simulink model "TubeMPC"  (Simulink 9.1)
settings: Solver=VariableStepAuto  StartTime=0.0  StopTime=40  FixedStep=0.1  RelTol=1e-3
undefined symbols (not defined in the file): ck_all, cx_all, cy_all, cyaw_all
libraries: Solver_SF x1, simulink x1
settings Model: Creator=MaoWenJie  LastModifiedBy=MaoWenJie
settings DataIOCC: SaveFormat=Dataset
settings OptimizationCC: LifeSpan=auto
settings DebuggingCC: UnderspecifiedInitializationDetection=Simplified  MergeDetectMultiDrivingBlocksExec=error  SFUnexpectedBacktrackingDiag=error  SFNoUnconditionalDefaultTransitionDiag=error  SFExecutionAtInitializationDiag=warning
settings HardwareCC: ProdBitPerPointer=64  ProdBitPerSizeT=64  ProdBitPerPtrDiffT=64  ProdLargestAtomicFloat=Float  ProdIntDivRoundTo=Zero  ProdEndianess=LittleEndian  ProdWordSize=64  ProdHWDeviceType=Intel->x86-64 (Windows64)
settings ModelReferenceCC: PropagateSignalLabelsOutOfModel=on
settings CodeAppCC: StateflowObjectComments=off
settings GRTTargetCC: TargetLangStandard=C99 (ISO)  CombineOutputUpdateFcns=on  GRTInterface=off
settings ConfigComp: CovMetricSettings=dwe  CovHtmlReporting=off  CovSaveCumulativeToWorkspaceVar=off  CovSaveSingleToWorkspaceVar=off  CovExternalEMLEnable=on

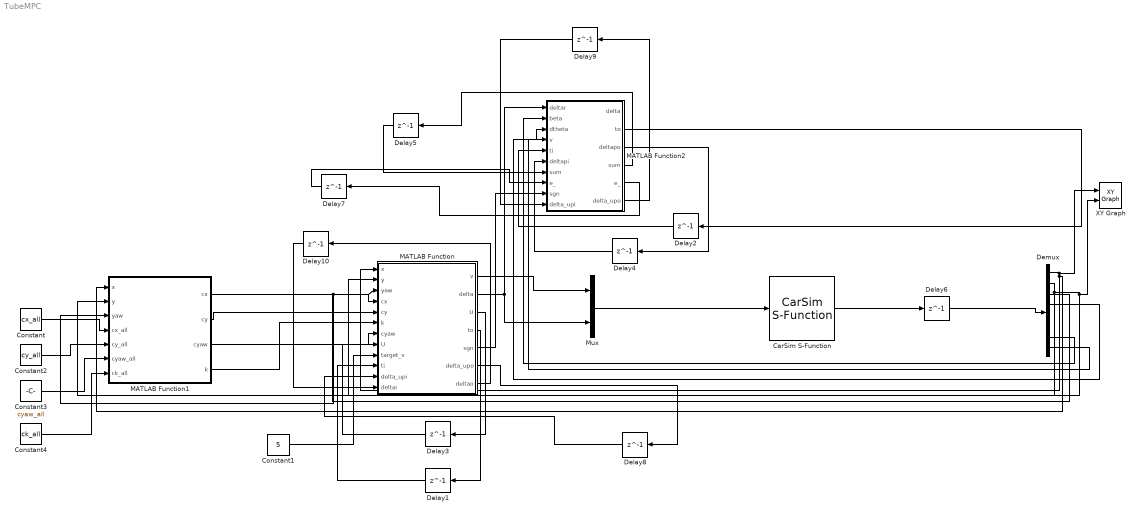
== system TubeMPC ==
  CarSim S-Function : Solver_SF/CarSim S-Function  Priority=3  SIMFILE=simfile.sim
  Constant : Constant  Value=cx_all
  Constant1 : Constant  Value=5
  Constant2 : Constant  Value=cy_all
  Constant3 : Constant  Value=cyaw_all
  Constant4 : Constant  Value=ck_all
  Delay{1..10} (10 alike) : Delay  DelayLength=1  InitialCondition=0
  Demux : Demux  Outputs=8
  MATLAB Function : MATLAB Function  Priority=2  InitFcn=|  TreatAsAtomicUnit=on
      | x = 0.1; y = -0.1; yaw = 0.1; 
      | U = [0.01;0.01];cx = 0.1;cy = -0.1;k = 1;cyaw = 1;ti = 0;
      | t = 0;
  MATLAB Function1 : MATLAB Function  Priority=1  TreatAsAtomicUnit=on
  MATLAB Function2 : MATLAB Function  InitFcn=ti = 0;deltapi = 0  TreatAsAtomicUnit=on
  Mux : Mux  Inputs=2
  XY Graph : simulink/Sinks/XY Graph  xmin=-1  xmax=200  ymin=-4  ymax=5  st=-1
  wires:
  Constant4/1 -> MATLAB Function1/7(ck_all)
  Constant3/1 -> MATLAB Function1/6(cyaw_all)
  Delay3/1 -> MATLAB Function/8("U ")
  Constant2/1 -> MATLAB Function1/5(cy_all)
  MATLAB Function1/1(cx) -> MATLAB Function/4(cx)
  MATLAB Function1/3(cyaw) -> MATLAB Function/7(cyaw)
  MATLAB Function/3(U) -> Delay3/1
  Constant/1 -> MATLAB Function1/4(cx_all)
  MATLAB Function1/4(k) -> MATLAB Function/6(k)
  Constant1/1 -> MATLAB Function/9(target_v)
  MATLAB Function1/2(cy) -> MATLAB Function/5(cy)
  CarSim S-Function/1 -> Delay6/1
  Delay6/1 -> Demux/1
  Demux/1 -> XY Graph/1, MATLAB Function1/1(x), MATLAB Function/1(x)
  Demux/2 -> XY Graph/2, MATLAB Function1/2(y), MATLAB Function/2(y)
  Demux/3 -> MATLAB Function1/3(yaw), MATLAB Function/3(yaw)
  MATLAB Function/1(v) -> Mux/1
  Mux/1 -> CarSim S-Function/1
  MATLAB Function/4(to) -> Delay1/1
  Delay1/1 -> MATLAB Function/10(ti)
  MATLAB Function/2(delta) -> Mux/2, MATLAB Function2/1(deltar)
  Demux/7 -> MATLAB Function2/2(beta)
  Demux/8 -> MATLAB Function2/3(dtheta)
  Demux/4 -> MATLAB Function2/4(v)
  MATLAB Function2/2(to) -> Delay2/1
  Delay2/1 -> MATLAB Function2/5(ti)
  MATLAB Function2/3(deltapo) -> Delay4/1
  Delay4/1 -> MATLAB Function2/6(deltapi)
  MATLAB Function2/4(sum) -> Delay5/1
  Delay5/1 -> MATLAB Function2/7("sum ")
  MATLAB Function2/5(e_) -> Delay7/1
  Delay7/1 -> MATLAB Function2/8("e_ ")
  MATLAB Function/5(sgn) -> MATLAB Function2/9(sgn)
  MATLAB Function/6(delta_upo) -> Delay8/1
  Delay8/1 -> MATLAB Function/11(delta_upi)
  MATLAB Function2/6(delta_upo) -> Delay9/1
  Delay9/1 -> MATLAB Function2/10(delta_upi)
  MATLAB Function/7(deltao) -> Delay10/1
  Delay10/1 -> MATLAB Function/12(deltai)

== matlab function MATLAB Function ==
  data: v output double; x input double; delta output double; y input double; yaw input double; cx input double; cy input double; k input double; cyaw input double; U input double size=2; target_v input double; U output double; ti input double; to output double; sgn output double; delta_upi input double; delta_upo output double; deltai input double; deltao output double
function    [v,delta,U,to,sgn,delta_upo,deltao] = ...
    tubeMpc_control(x,y,yaw,cx,cy,k,cyaw,U,target_v,ti,delta_upi,deltai) 
coder.extrinsic('dlqr');
coder.extrinsic('optimoptions');
coder.extrinsic('quadprog');
Length = 2.6;
yaw = yaw*pi/180;
u = [x,y,yaw];
vd1=target_v ;
vd2=atan(Length * k);
dt = 0.4;



if ti == 0
r = [cx, cy, cyaw];
    Nx=3;%状态量的个数
    Nu =2;%控制量的个数
    Np =60;%预测步长
    Nc=30;%控制步长
    Row=10;%松弛因子
    Q=100*eye(Nx*Np,Nx*Np);    
    R=1*eye(Nc*Nu);
    t_d =r(3);%角度为弧度
    
    kesi=zeros(Nx+Nu,1);
    kesi(1)=u(1)-r(1);%u(1)==X(1)
    kesi(2)=u(2)-r(2);%u(2)==X(2)
    kesi(3)=u(3)-r(3); %u(3)==X(3)
    kesi(4)=U(1);
    kesi(5)=U(2);
%     fprintf('Update start, u(1)=%4.2f\n',U(1))
%     fprintf('Update start, u(2)=%4.2f\n',U(2))
    T=dt;
    % Mobile Robot Parameters
    L = Length;
    % Mobile Robot variable
    
%矩阵初始化   
    delta_u=zeros(Nx,Nu);
    
    a=[1    0   -vd1*sin(t_d)*T;
       0    1   vd1*cos(t_d)*T;
       0    0   1;];
    b=[cos(t_d)*T   0;
       sin(t_d)*T   0;
       tan(vd2)*T/L      vd1*T/(L * (cos(vd2)^2))];
    A = zeros(Nu+Nx,Nu+Nx);
    A(1:Nx,1:Nx)=a;
    A(1:Nx,Nx+1:Nx+Nu)=b;
    A(Nx+1:Nx+Nu,Nx+1:Nx+Nu) = eye(Nu);
    B = ones(Nx+Nu,Nu);
    B(1:Nx,:)=b;
    B(Nx+1:Nx+Nu,:)=eye(Nu);
    C=[1 0 0 0 0;0 1 0 0 0;0 0 1 0 0;];
    Px = zeros(Nx*Np,Nx+Nu);
    Hx = zeros(Nx*Np,Nu*Nc);
    for j=1:1:Np
        Px(1+(j-1)*Nx:j*Nx,:)=C*A^j;
        for k=1:1:Nc
            if k<=j
                Hx(1+(j-1)*Nx:j*Nx,1+(k-1)*Nu:k*Nu)=C*A^(j-k)*B;
            else 
                Hx(1+(j-1)*Nx:j*Nx,1+(k-1)*Nu:k*Nu)=zeros(Nx,Nu);
            end
        end
    end
    theta = [eye(Nx+Nu),zeros(Nx+Nu,Nu*Nc)];
    xi = [zeros(Nu*Nc,Nx+Nu),eye(Nu*Nc)];
    H=[theta'*Px'*Q*Px*theta+xi'*Hx'*Q*Px*theta+theta'*Px'*Q*Hx*xi+xi'*Hx'*Q*Hx*xi+xi'*R*xi,zeros(Nu*Nc+Nx+Nu,1);
        zeros(1,Nu*Nc+Nx+Nu),Row];
    H = (H+H')/2;
    f=[];
    
 %% 以下为约束生成区域
 %不等式约束
    A_t=zeros(Nc,Nc);%见falcone论文 P181
    for p=1:1:Nc
        for q=1:1:Nc
            if q<=p 
                A_t(p,q)=1;
            else 
                A_t(p,q)=0;
            end
        end 
    end 
    A_I=kron(A_t,eye(Nu));%对应于falcone论文约束处理的矩阵A,求克罗内克积
    Ut=kron(ones(Nc,1),U);%此处感觉论文里的克罗内科积有问题,暂时交换顺序
    umin=[0;-0.64];%维数与控制变量的个数相同
    umax=[20;0.64];
    w = 0;
    wmax = [w;w;0;0;0];
    wmin = [-w;-w;0;0;0];
    Q_ = eye(5);
    R_ = eye(2);
    Kp = zeros(Nu,Nu+Nx);
    Kp = dlqr(A,B,Q_,R_);
    Kp = -Kp;
    Ak = zeros(Nx+Nu,Nx+Nu);
    Ak = A+B*Kp;
    aphl1 = sqrt(Ak(3,1)^2+Ak(3,2)^2);
    aphl2 = sqrt(Ak(4,1)^2+Ak(4,2)^2);
    aphl3 = sqrt(Ak(5,1)^2+Ak(5,2)^2);
    w = 0.7*w;
    wmax(3:5)=[aphl1*w;aphl2*w;aphl3*w];
    wmin(3:5)=-wmax(3:5);
    delta_umin = [ -2.2 ; -0.64];
    delta_umax = [  2.2 ;  0.64];
    delta_Umin=kron(ones(Nc,1),delta_umin);
    delta_Umax=kron(ones(Nc,1),delta_umax);
    Umin=kron(ones(Nc,1),umin);
    Umax=kron(ones(Nc,1),umax);
    M = 10;
    A_cons=[A_I*xi zeros(Nu*Nc,1);-A_I*xi zeros(Nu*Nc,1)];
    b_cons=[Umax-Ut;-Umin+Ut];
   % 状态量约束
    lb=[kesi-wmax;delta_Umin;0];%（求解方程）状态量下界，包含控制时域内控制增量和松弛因子
    ub=[kesi-wmin;delta_Umax;M];%（求解方程）状态量上界，包含控制时域内控制增量和松弛因子

    %% 开始求解过程
    u_ = zeros(Nu*Nc,1);
    x_ = zeros(Nx+Nu,1);
    kk = zeros(Nu,1);
    delta_u = zeros(Nu,1);
    exitflag = 0;
    options = optimoptions('quadprog','Display','iter','MaxIterations',100,'TolFun',1e-16);
    [X,fval,exitflag]=quadprog(H,f,A_cons,b_cons,[],[],lb,ub,[],options);
    %% 计算输出
    if exitflag==-2
    delta_u(1)=0;
    delta_u(2)=randn(1)*0.001;
    else
    u_ = xi*X(1:(Nu*Nc+Nx+Nu));
    x_ = theta*X(1:(Nu*Nc+Nx+Nu));
    kk = u_(1:2)+Kp*(kesi-x_);
    delta_u(1)=kk(1);
    delta_u(2)=kk(2);
    end
    U(1)=kesi(4)+delta_u(1) ;%用于存储上一个时刻的控制量
    U(2)=kesi(5)+delta_u(2); %kesi here is previous step U
    v=U(1)+vd1; %  vd1 and vd2 here is U_ref
    delta=U(2)+vd2;
    delta_upo = delta;
else
    delta_upo = delta_upi;
end
if ti == 99
    ti = -1;
    sgn = 1;
    v  = target_v;
    v = v*3.6;
    delta = delta_upi;
    delta = delta*180/pi;
    deltao = delta;
else
    sgn = 0;
    v  = target_v;
    v = v*3.6;
    delta = deltai;
    deltao = deltai;
end
to  = ti+1;
end

== matlab function MATLAB Function2 ==
  data: deltar input double; delta output double; beta input double; dtheta input double; v input double; ti input double; to output double; deltapi input double; deltapo output double; sum input double; e_ input double; sgn input double; sum output double; e_ output double; delta_upi input double; delta_upo output double
function [delta,to,deltapo,sum,e_,delta_upo] = PID_control(deltar,beta,dtheta,v,ti,deltapi,sum,e_,sgn,delta_upi)
if sgn == 1
    sum = 0;
end
    
if ti==0
Kp1 = 0;
Kp2 = 1;
Ki2 = 0;
Kd2 = 0;
dr = 1.56;
df = 1.04;
deltar = deltar*pi/180;
beta = beta*pi/180;
dtheta = dtheta*pi/180;

betar = atan(dr*tan(deltar)/(df+dr));
dthetar = v*cos(betar)*tan(deltar)/(dr+df);
e = dthetar-dtheta;
if sgn == 1
    e_=e;
end
sum = sum+e;
delta = Kp1*(betar-beta)+Kp2*(dthetar-dtheta)+Ki2*sum+Kd2*(e-e_);
e_ = e;
delta_upo = delta;
%delta = deltar*180/pi;
%deltar = deltar*180/pi;
else
delta_upo = delta_upi;
end
if ti == 19
ti = -1;
delta = delta_upi;
delta = delta*180/pi;
deltapo = delta;
else
delta = deltapi;
deltapo = deltapi;
end
%delta = deltar;
to = ti+1;

== matlab function MATLAB Function1 ==
  data: x input double; cx output double; y input double; yaw input double; cx_all input double; cy_all input double; cyaw_all input double; ck_all input double; cy output double; cyaw output double; k output double
function [cx,cy,cyaw,k] = calc_target_index(x,y,yaw, cx_all,cy_all,cyaw_all,ck_all)% find my location, and lateral error
N =  length(cx_all);
Distance = zeros(N,1);
L=2.6;
% K = v*tan(delta)/L;
% x = x + v*(cos(yaw)-cos(yaw+K*T))/K;
% y = y + v*(sin(yaw+K*T)-sin(yaw))/K;
for i = 1:N
Distance(i) =  sqrt((cx_all(i)-x)^2 + (cy_all(i)-y)^2 );
end
[value, location]= min(Distance);
ind  = location;
cx = cx_all(ind);
cy = cy_all(ind);
cyaw = cyaw_all(ind);
k = ck_all(ind);
end
